simulink model "scen2_PDproposed"  (R2021b)
settings: Solver=ode4  StartTime=0.0  StopTime=tsim+1  FixedStep=sampleRate  RelTol=1e-3
undefined symbols (not defined in the file): alpha, des_x, des_y, des_z, Kd, Kdz, Kp, Kpz, peak_mp, Q, saturation_on, t_end_mp
libraries: dspmtrx3 x1
settings Model: Creator=PC  LastModifiedBy=kangm
settings SolverCC: AlgebraicLoopSolver=TrustRegion
settings DataIOCC: ReturnWorkspaceOutputs=off
settings DebuggingCC: SFMachineParentedDataDiag=warning

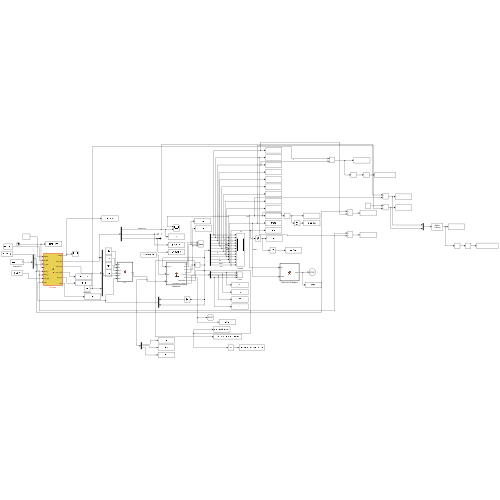
[thumbnail: Simulink's stored preview of the top-level diagram]
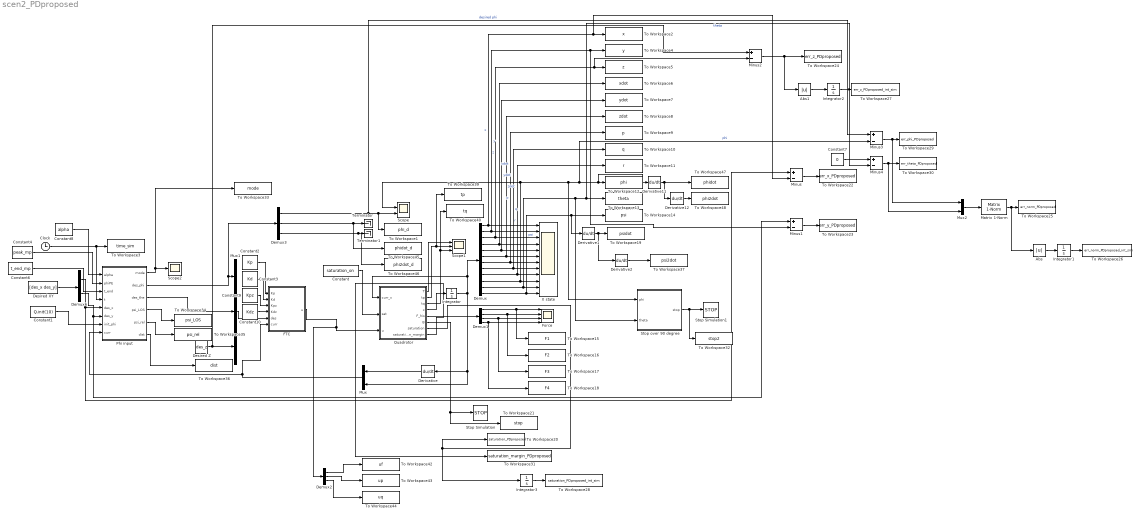
== system scen2_PDproposed ==
  Abs : Abs
  Abs1 : Abs
  Clock : Clock
  Constant : Constant  Value=saturation_on
  Constant1 : Constant  Value=Q.init(10)
  Constant10 : Constant  Value=Kdz
  Constant2 : Constant  Value=Kp
  Constant3 : Constant  Value=Kd
  Constant4 : Constant  Value=peak_mp
  Constant6 : Constant  Value=t_end_mp
  Constant7 : Constant  Value=0
  Constant8 : Constant  Value=alpha
  Constant9 : Constant  Value=Kpz
  Demux : Demux  Outputs=12
  Demux1 : Demux
  Demux2 : Demux  Outputs=3
  Demux3 : Demux  Outputs=3
  Demux6 : Demux  Outputs=2
  Derivative{,1..2,11..12} (5 alike) : Derivative
  Desired XY : Constant  Value=[des_x des_y]
  Desired Z : Constant  Value=des_z
  FTC : MATLAB Function  TreatAsAtomicUnit=on
  Force : Scope  NumInputPorts=4
  Integrator : Integrator  InitialCondition=Q.init
  Integrator1 : Integrator
  Integrator2 : Integrator
  Integrator3 : Integrator
  Matrix 1-Norm : dspmtrx3/Matrix  1-Norm  roundingMode=Floor  overflowMode=off  outputDataTypeStr=Inherit: Same as accumulator  outputMin=[]  outputMax=[]  outputLastDataTypeStr=Inherit: Same as accumulator
      settings: SourceProductBaseCode=DS
  Minus{,1..4} (5 alike) : Sum  Inputs=+-
  Mux : Mux  Inputs=2
  Mux1 : Mux  Inputs=3
  Mux2 : Mux  Inputs=2
  Phi input : MATLAB Function  TreatAsAtomicUnit=on
  Quadrotor : MATLAB Function  TreatAsAtomicUnit=on
  Scope : Scope  NumInputPorts=2
  Scope1 : Scope  NumInputPorts=3
  Scope2 : Scope
  Stop Simulation : Stop
  Stop Simulation1 : Stop
  Stop over 90 degree : MATLAB Function  TreatAsAtomicUnit=on
  Terminator : Terminator
  Terminator1 : Terminator
  To Workspace1 : ToWorkspace  VariableName=phi_d  SampleTime=-1
      settings: Save2DSignal=2-D array (concatenate along first dimension)
  To Workspace10 : ToWorkspace  VariableName=q  SampleTime=-1
      settings: Save2DSignal=2-D array (concatenate along first dimension)
  To Workspace11 : ToWorkspace  VariableName=r  SampleTime=-1
      settings: Save2DSignal=2-D array (concatenate along first dimension)
  To Workspace12 : ToWorkspace  VariableName=phi  SampleTime=-1
      settings: Save2DSignal=2-D array (concatenate along first dimension)
  To Workspace13 : ToWorkspace  VariableName=theta  SampleTime=-1
      settings: Save2DSignal=2-D array (concatenate along first dimension)
  To Workspace14 : ToWorkspace  VariableName=psi  SampleTime=-1
      settings: Save2DSignal=2-D array (concatenate along first dimension)
  To Workspace15 : ToWorkspace  VariableName=F1  SampleTime=-1
      settings: Save2DSignal=2-D array (concatenate along first dimension)
  To Workspace16 : ToWorkspace  VariableName=F2  SampleTime=-1
      settings: Save2DSignal=2-D array (concatenate along first dimension)
  To Workspace17 : ToWorkspace  VariableName=F3  SampleTime=-1
      settings: Save2DSignal=2-D array (concatenate along first dimension)
  To Workspace18 : ToWorkspace  VariableName=F4  SampleTime=-1
      settings: Save2DSignal=2-D array (concatenate along first dimension)
  To Workspace19 : ToWorkspace  VariableName=psidot  SampleTime=-1
      settings: Save2DSignal=2-D array (concatenate along first dimension)
  To Workspace2 : ToWorkspace  VariableName=x  SampleTime=-1
      settings: Save2DSignal=2-D array (concatenate along first dimension)
  To Workspace20 : ToWorkspace  VariableName=saturation_PDproposed  SampleTime=-1
      settings: Save2DSignal=2-D array (concatenate along first dimension)
  To Workspace21 : ToWorkspace  VariableName=stop  SampleTime=-1
      settings: Save2DSignal=2-D array (concatenate along first dimension)
  To Workspace22 : ToWorkspace  VariableName=err_x_PDproposed  SampleTime=-1
      settings: Save2DSignal=2-D array (concatenate along first dimension)
  To Workspace23 : ToWorkspace  VariableName=err_y_PDproposed  SampleTime=-1
      settings: Save2DSignal=2-D array (concatenate along first dimension)
  To Workspace24 : ToWorkspace  VariableName=err_z_PDproposed  SampleTime=-1
      settings: Save2DSignal=2-D array (concatenate along first dimension)
  To Workspace25 : ToWorkspace  VariableName=err_norm_PDproposed  SampleTime=-1
      settings: Save2DSignal=2-D array (concatenate along first dimension)
  To Workspace26 : ToWorkspace  VariableName=err_norm_PDproposed_int_sim  SampleTime=-1
      settings: Save2DSignal=2-D array (concatenate along first dimension)
  To Workspace27 : ToWorkspace  VariableName=err_z_PDproposed_int_sim  SampleTime=-1
      settings: Save2DSignal=2-D array (concatenate along first dimension)
  To Workspace28 : ToWorkspace  VariableName=saturation_PDproposed_int_sim  SampleTime=-1
      settings: Save2DSignal=2-D array (concatenate along first dimension)
  To Workspace29 : ToWorkspace  VariableName=err_phi_PDproposed  SampleTime=-1
      settings: Save2DSignal=2-D array (concatenate along first dimension)
  To Workspace3 : ToWorkspace  VariableName=time_sim  SampleTime=-1
      settings: Save2DSignal=2-D array (concatenate along first dimension)
  To Workspace30 : ToWorkspace  VariableName=err_theta_PDproposed  SampleTime=-1
      settings: Save2DSignal=2-D array (concatenate along first dimension)
  To Workspace31 : ToWorkspace  VariableName=saturation_margin_PDproposed  SampleTime=-1
      settings: Save2DSignal=2-D array (concatenate along first dimension)
  To Workspace32 : ToWorkspace  VariableName=stop2  SampleTime=-1
      settings: Save2DSignal=2-D array (concatenate along first dimension)
  To Workspace33 : ToWorkspace  VariableName=mode  SampleTime=-1
      settings: Save2DSignal=2-D array (concatenate along first dimension)
  To Workspace34 : ToWorkspace  VariableName=psi_LOS  SampleTime=-1
      settings: Save2DSignal=2-D array (concatenate along first dimension)
  To Workspace35 : ToWorkspace  VariableName=psi_rel  SampleTime=-1
      settings: Save2DSignal=2-D array (concatenate along first dimension)
  To Workspace36 : ToWorkspace  VariableName=dist  SampleTime=-1
      settings: Save2DSignal=2-D array (concatenate along first dimension)
  To Workspace37 : ToWorkspace  VariableName=psi2dot  SampleTime=-1
      settings: Save2DSignal=2-D array (concatenate along first dimension)
  To Workspace39 : ToWorkspace  VariableName=tp  SampleTime=-1
      settings: Save2DSignal=2-D array (concatenate along first dimension)
  To Workspace4 : ToWorkspace  VariableName=y  SampleTime=-1
      settings: Save2DSignal=2-D array (concatenate along first dimension)
  To Workspace40 : ToWorkspace  VariableName=tq  SampleTime=-1
      settings: Save2DSignal=2-D array (concatenate along first dimension)
  To Workspace42 : ToWorkspace  VariableName=uf  SampleTime=-1
      settings: Save2DSignal=2-D array (concatenate along first dimension)
  To Workspace43 : ToWorkspace  VariableName=up  SampleTime=-1
      settings: Save2DSignal=2-D array (concatenate along first dimension)
  To Workspace44 : ToWorkspace  VariableName=uq  SampleTime=-1
      settings: Save2DSignal=2-D array (concatenate along first dimension)
  To Workspace45 : ToWorkspace  VariableName=phidot_d  SampleTime=-1
      settings: Save2DSignal=2-D array (concatenate along first dimension)
  To Workspace46 : ToWorkspace  VariableName=phi2dot_d  SampleTime=-1
      settings: Save2DSignal=2-D array (concatenate along first dimension)
  To Workspace47 : ToWorkspace  VariableName=phidot  SampleTime=-1
      settings: Save2DSignal=2-D array (concatenate along first dimension)
  To Workspace48 : ToWorkspace  VariableName=phi2dot  SampleTime=-1
      settings: Save2DSignal=2-D array (concatenate along first dimension)
  To Workspace5 : ToWorkspace  VariableName=z  SampleTime=-1
      settings: Save2DSignal=2-D array (concatenate along first dimension)
  To Workspace6 : ToWorkspace  VariableName=xdot  SampleTime=-1
      settings: Save2DSignal=2-D array (concatenate along first dimension)
  To Workspace7 : ToWorkspace  VariableName=ydot  SampleTime=-1
      settings: Save2DSignal=2-D array (concatenate along first dimension)
  To Workspace8 : ToWorkspace  VariableName=zdot  SampleTime=-1
      settings: Save2DSignal=2-D array (concatenate along first dimension)
  To Workspace9 : ToWorkspace  VariableName=p  SampleTime=-1
      settings: Save2DSignal=2-D array (concatenate along first dimension)
  X state : Scope  NumInputPorts=12
  wires:
  Quadrotor/4(x) -> Integrator/1
  Mux1/1 -> FTC/5(des)
  Integrator/1 -> Demux/1, Quadrotor/1(curr_x), Derivative/1, Mux/2
  Demux/1 -> Minus/2, To Workspace2/1, X state/1  "x"
  Demux/2 -> Minus1/2, To Workspace4/1, X state/2  "y"
  Demux/4 -> To Workspace6/1, X state/4  "xdot"
  Demux/5 -> To Workspace7/1, X state/5  "ydot"
  Demux/6 -> To Workspace8/1, X state/6  "zdot"
  Demux/7 -> To Workspace9/1, X state/7  "p"
  Demux/8 -> To Workspace10/1, X state/8  "q"
  Demux/9 -> To Workspace11/1, X state/9  "r"
  Mux/1 -> FTC/6(curr), Phi input/8(curr)
  Derivative/1 -> Mux/1
  Clock/1 -> Phi input/4(t), To Workspace3/1
  Demux6/1 -> Minus/1, Phi input/5(des_x)
  Desired XY/1 -> Demux6/1
  Quadrotor/5(F_his) -> Demux1/1
  Demux1/1 -> Force/1, To Workspace15/1
  Demux1/3 -> Force/3, To Workspace17/1
  Demux1/4 -> Force/4, To Workspace18/1
  Demux1/2 -> Force/2, To Workspace16/1
  Demux/12 -> Derivative1/1, To Workspace14/1, X state/12  "psi"
  Derivative1/1 -> Derivative2/1, To Workspace19/1
  Constant/1 -> Quadrotor/2(sat)
  Demux3/3 -> To Workspace46/1, Terminator1/1
  Constant1/1 -> Phi input/7(init_phi)
  Phi input/2(des_phi) -> Demux3/1, Mux1/1
  Phi input/3(des_the) -> Mux1/2
  Constant6/1 -> Phi input/3(t_end)
  Constant4/1 -> Phi input/2(phiPE)
  Constant2/1 -> FTC/1(Kp)
  Constant3/1 -> FTC/2(Kd)
  Quadrotor/1(T) -> Scope1/1
  Quadrotor/6(B) -> To Workspace21/1, Stop Simulation/1
  Quadrotor/7(saturation) -> To Workspace20/1, Integrator3/1
  Integrator3/1 -> To Workspace28/1
  Demux/3 -> Minus2/2, To Workspace5/1, X state/3  "z"
  Minus1/1 -> To Workspace23/1
  Demux6/2 -> Minus1/1, Phi input/6(des_y)
  Matrix 1-Norm/1 -> Abs/1, To Workspace25/1
  Demux3/1 -> To Workspace1/1, Scope/2, Minus3/1  "desired phi"
  Mux2/1 -> Matrix 1-Norm/1
  Desired Z/1 -> Minus2/1, Mux1/3
  Abs/1 -> Integrator1/1
  Integrator1/1 -> To Workspace26/1
  Abs1/1 -> Integrator2/1
  Integrator2/1 -> To Workspace27/1
  Minus/1 -> To Workspace22/1
  Minus2/1 -> Abs1/1, To Workspace24/1
  Minus3/1 -> Mux2/1, To Workspace29/1
  Minus4/1 -> Mux2/2, To Workspace30/1
  Constant7/1 -> Minus4/1
  Demux/10 -> Stop over 90 degree/1(phi), Minus3/2, Derivative11/1, To Workspace12/1, Scope/1, X state/10  "phi"
  Stop over 90 degree/1(stop) -> To Workspace32/1, Stop Simulation1/1
  Demux/11 -> Stop over 90 degree/2(theta), Minus4/2, To Workspace13/1, X state/11  "theta"
  Quadrotor/8(saturation_margin) -> To Workspace31/1
  Phi input/1(mode) -> To Workspace33/1, Scope2/1
  Derivative2/1 -> To Workspace37/1
  Demux3/2 -> To Workspace45/1, Terminator/1
  Phi input/4(psi_LOS) -> To Workspace34/1
  Phi input/5(psi_rel) -> To Workspace35/1
  Phi input/6(dist) -> To Workspace36/1
  Quadrotor/3(tq) -> To Workspace40/1, Scope1/3
  Quadrotor/2(tp) -> To Workspace39/1, Scope1/2
  Demux2/3 -> To Workspace44/1
  Demux2/2 -> To Workspace43/1
  Demux2/1 -> To Workspace42/1
  FTC/1(u) -> Demux2/1, Quadrotor/3(u)
  Derivative11/1 -> Derivative12/1, To Workspace47/1
  Derivative12/1 -> To Workspace48/1
  Constant8/1 -> Phi input/1(alpha)
  Constant10/1 -> FTC/4(Kdz)
  Constant9/1 -> FTC/3(Kpz)

== matlab function scen2_PDproposed/FTC ==
  data: Kp input; Kd input; Kpz input; Kdz input; des input; u output; curr input
function u   = pd(Kp,Kd,Kpz,Kdz,des,curr)

m = 1.282; g = 9.81;
Ix = 4.856*10^-3; Iy = Ix; Iz = 8.801*10^-3;
b = 0.0066;
kr = 0.02; %drag coefficient
kt = 0.5;
% kt = 0.25;
l = 0.1;

% current state
N = 0;
xdot   = curr(N+1); ydot   = curr(N+2); zdot   = curr(N+3);
x2dot  = curr(N+4); y2dot  = curr(N+5); z2dot  = curr(N+6);
pdot   = curr(N+7); qdot   = curr(N+8); rdot   = curr(N+9);
phidot = curr(N+10);thedot = curr(N+11);psidot = curr(N+12);

N = 12;
x    = curr(N+1); y    = curr(N+2); z    = curr(N+3);
xdot = curr(N+4); ydot = curr(N+5); zdot = curr(N+6);
p    = curr(N+7); q    = curr(N+8); r    = curr(N+9);
phi  = curr(N+10);the  = curr(N+11);psi  = curr(N+12);
des_temp = zeros(7,1);
des_temp = des;
des = des_temp;
% desired state
phi_d = des(1);
phidot_d = des(2);
phi2dot_d = des(3);
the_d = des(4);
thedot_d = des(5);
the2dot_d = des(6);
z_d   = des(7);


% Feedback PD Control
% phi
% phi2dot = f1(~~)+1/Ix*tp

% Kp = 3;
% Kd = 4;

% Kp = 100;
% Kd = 1;

F = [p + q*sin(phi)*tan(the) + r*cos(phi)*tan(the)
     q*cos(phi) - r*sin(phi)
     -(Iz - Iy)*q*r/Ix
     -(Ix - Iz)*p*r/Iy
     -kr*r/Iz
     zdot
     -kt*zdot/m - g];
 
G = [0 0 0
     0 0 0
     0 1/Ix 0
     0 0 1/Iy
     b/Iz -2*b/(l*Iz) 0
     0 0 0
     cos(phi)*cos(the)/m 0 0];
 
J = [q*cos(phi)*tan(the)-r*sin(phi)*tan(the) q*sin(phi)*sec(the)^2+r*cos(phi)*sec(the)^2 1 sin(phi)*tan(the) cos(phi)*tan(the) 0 0
     -q*sin(phi)-r*cos(phi) 0 0 cos(phi) -sin(phi) 0 0
     0 0 0 0 0 0 1];

ubar = [phi2dot_d + Kp*(phi_d-phi) + Kd*(phidot_d-phidot)
        the2dot_d + Kp*(the_d-the) + Kd*(thedot_d-thedot)
        Kpz*(z_d-z) + Kdz*(0-zdot)];
    
u = inv(J*G)*(-J*F + ubar);

% u = [12.5813 0.0013 0]';
% u = [13.3835 0.0259 0]';

% tp = u_prev(1);
% tq = u_prev(2);
% T = u_prev(3);

 
% f1 = qdot*sin(phi)*tan(the) + q*cos(phi)*phidot*tan(the) + q*sin(phi)*1/cos(the)^2*thedot...
%     + rdot*cos(phi)*tan(the) + r*(-sin(phi)*phidot)*tan(the) + r*cos(phi)*1/cos(the)^2*thedot ...
%     + (Ix-Iz)/Ix*q*r;
% 
% % tp = Ix*(-f1+ 3*(phi_d-phi) + 4*(phidot_d-phidot));
% tp = Ix*(-f1+ Kp*(phi_d-phi) + Kd*(phidot_d-phidot));
% 
% 
% %theta
% %the2dot = g1(~~) + cos(phi)/Ix * tq
% h1 = -q*sin(phi)*phidot-rdot*sin(phi)-r*cos(phi)*phidot ...
%     + (Iz-Ix)/Ix*p*r*cos(phi);
% % tq = Ix*(-h1+ 3*(the_d-the) + 5*(thedot_d-thedot));
% tq = Ix*(-h1+ Kp*(the_d-the) + Kd*(thedot_d-thedot));
% 
% %z
% T = m/(cos(the)*cos(phi))*(g + 3*(z_d-z) + (0-zdot));

% u = [T tp tq]';

== matlab function scen2_PDproposed/Quadrotor ==
  data: T output; tp output; tq output; curr_x input; sat input; u input; x output; F_his output; B output; saturation output; saturation_margin output
function [T,tp,tq,x,F_his,B,saturation,saturation_margin] = system(curr_x,sat,u)
% x = {xyz xyzvel pqr phi theta psi}
x = zeros(12,1);
% Properties
m = 1.282; g = 9.81;
Ix = 4.856*10^-3; Iy = Ix; Iz = 8.801*10^-3;
b = 0.0066;
kr = 0.02;
kt = 0.5;
l = 0.1;

u_temp = zeros(3,1);
u_temp = u;
u = u_temp;

T = u(1); tp = u(2); tq = u(3);% tr = u(4);
tr = b*(T-2*tp/l);
A = [1 1 1; 0 l 0;-l 0 l];

F=inv(A)*[T tp tq]';

f1 = F(1); f2 = F(2); f3 = F(3);
ub = m*g;
lb = 0;

saturation1_lb = 0;
saturation1_ub = 0;
saturation2_lb = 0;
saturation2_ub = 0;
saturation3_lb = 0;
saturation3_ub = 0;
saturation1_lb_margin = 0;
saturation1_ub_margin = 0;
saturation2_lb_margin = 0;
saturation2_ub_margin = 0;
saturation3_lb_margin = 0;
saturation3_ub_margin = 0;

if sat == 1
    if f1 < lb
        saturation1_lb = abs(lb - f1);
        saturation1_lb_margin = abs(lb - f1);
        f1 = lb;
    else
        saturation1_lb_margin = lb - f1;
    end
    
    if f1 > ub
        saturation1_ub = abs(ub - f1);
        saturation1_ub_margin = abs(ub - f1);
        f1 = ub;
    else
        saturation1_ub_margin = f1 - ub;
    end
    
    if f2 < lb
        saturation2_lb = abs(lb - f2);
        saturation2_lb_margin = abs(lb - f2);
        f2 = lb;
    else
        saturation2_lb_margin = lb - f2;
    end
    
    if f2 > ub
        saturation2_ub = abs(ub - f2);
        saturation2_ub_margin = abs(ub - f2);
        f2 = ub;
    else
        saturation2_ub_margin = f2 - ub;
    end
    
    if f3 < lb
        saturation3_lb = abs(lb - f3);
        saturation3_lb_margin = abs(lb - f3);
        f3 = lb;
    else
        saturation3_lb_margin = lb - f3;
    end
    
    if f3 > ub
        saturation3_ub = abs(ub - f3);
        saturation3_ub_margin = abs(ub - f3);
        f3 = ub;
    else
        saturation3_ub_margin = f3 - ub;
    end
end

saturation = max([saturation1_lb,saturation1_ub,saturation2_lb,saturation2_ub,saturation3_lb,saturation3_ub]);
saturation_margin = max([saturation1_lb_margin,saturation1_ub_margin,saturation2_lb_margin,saturation2_ub_margin,saturation3_lb_margin,saturation3_ub_margin]);

f4 = 0;
F_his = [f1 f2 f3 f4]';
T = f1+f2+f3;
tp = l*(f2);
tq = l*(f3-f1);
tr = b*(f1+f3-f2);

% Current state
x1  = curr_x(1);
x2  = curr_x(2);
x3  = curr_x(3);
x4  = curr_x(4);
x5  = curr_x(5);
x6  = curr_x(6);
x7  = curr_x(7);
x8  = curr_x(8);
x9  = curr_x(9);
x10 = curr_x(10);
x11 = curr_x(11);
x12 = curr_x(12);

% Position
x(1) = x4;
x(2) = x5;
x(3) = x6;
% Velocity
x(4) = T/m*(cos(x12)*sin(x11)*cos(x10) + sin(x12)*sin(x10)) - kt/m*x4;
x(5) = T/m*(sin(x12)*sin(x11)*cos(x10) - cos(x12)*sin(x10)) - kt/m*x5;
x(6) = -g + T*(1/m)*(cos(x10)*cos(x11)) - kt/m*x6;
% Body rate
x(7) = ((Ix-Iz)*x8*x9 + tp)/Ix;
x(8) = ((Iz-Ix)*x7*x9 + tq)/Ix;
x(9) = (-kr*x9 + tr)/Iz;
% Angle
x(10) = x7 + x8*sin(x10)*tan(x11) + x9*cos(x10)*tan(x11);
x(11) = x8*cos(x10) - x9*sin(x10);
x(12) = x8*sin(x10)/cos(x11) + x9*cos(x10)*cos(x11);

if x3<=0
    B=1;
else
    B=0;
end

== matlab function scen2_PDproposed/Stop over 90 degree ==
  data: phi input; stop output; theta input
function stop = fcn(phi, theta)

stop = 0;
max_attitude = deg2rad(90);

if abs(phi) >= max_attitude || abs(theta) >= max_attitude
    stop = 1;
end

== matlab function scen2_PDproposed/Phi input ==
  settings: updateMethod=DISCRETE
  data: alpha input; mode output; phiPE input; t_end input; des_phi output; des_the output; t input; des_x input; des_y input; init_phi input; curr input; psi_LOS output; psi_rel output; dist output
function [mode,des_phi,des_the,psi_LOS,psi_rel,dist]  = fcn(alpha,phiPE,t_end,t,des_x,des_y,init_phi,curr)

m = 1.282; g = 9.81;
Ix = 4.856*10^-3; Iz = 8.801*10^-3; Iy = Ix; I = (Iz-Iy)/Ix;
b = 0.0066;
kr = 0.02; %drag coefficient
kt = 0.5;
l = 0.1;

phi0 = init_phi;
T = t_end;

rPE = (-kr/b+sqrt((kr/b)^2+8*m*g/(l*cos(phiPE))*(Iz-Iy)*tan(phiPE)))/(4*(Iz-Iy)*tan(phiPE)/l);
psidotPE = rPE*(tan(phiPE)*sin(phiPE)+cos(phiPE)); 
TPE = 2*pi/psidotPE;

phiPE2 = phiPE - alpha;
rPE2 = (-kr/b+sqrt((kr/b)^2+8*m*g/(l*cos(phiPE2))*(Iz-Iy)*tan(phiPE2)))/(4*(Iz-Iy)*tan(phiPE2)/l);
psidotPE2 = rPE2*(tan(phiPE2)*sin(phiPE2)+cos(phiPE2)); 
TPE2 = 2*pi/psidotPE2;

fPE2 = 1/TPE2;
fPE2 = fPE2*1.0004;
toff = 1/(4*fPE2);

a0 = phi0;
a1 = 0;
a2 = 0;
a3 = - (10*phi0 - 10*phiPE)/T^3;
a4 = (15*phi0 - 15*phiPE)/T^4;
a5 = -(6*phi0 - 6*phiPE)/T^5;

% current state
N = 0;
xdot   = curr(N+1); ydot   = curr(N+2); zdot   = curr(N+3);
x2dot  = curr(N+4); y2dot  = curr(N+5); z2dot  = curr(N+6);
pdot   = curr(N+7); qdot   = curr(N+8); rdot   = curr(N+9);
phidot = curr(N+10);thedot = curr(N+11);psidot = curr(N+12);

N = 12;
x    = curr(N+1); y    = curr(N+2); z    = curr(N+3);
xdot = curr(N+4); ydot = curr(N+5); zdot = curr(N+6);
p    = curr(N+7); q    = curr(N+8); r    = curr(N+9);
phi  = curr(N+10);the  = curr(N+11);psi  = curr(N+12);

while psi > pi
    psi = psi - 2*pi;
end

while psi < -pi
    psi = psi + 2*pi;
end

R = 0.2016;

C_x = des_x;
C_y = des_y;
x_d = -R*sin(psi) + C_x; y_d = R*cos(psi) + C_y;
xdot_d = -R*cos(psi)*psidot; ydot_d = -R*sin(psi)*psidot;

dist = sqrt((x_d-x)^2+(y_d-y)^2);

psi_LOS = atan2(des_y-y,des_x-x);

psi_rel = psi_LOS - psi;
while psi_rel > pi
    psi_rel = psi_rel - 2*pi;
end

while psi_rel < -pi
    psi_rel = psi_rel + 2*pi;
end

kp = 1; kd = 1.5;

persistent x0 y0 psi0 psi_LOS0 xPSMP yPSMP psiPSMP tPSMP tauPSMP 
if isempty(x0)
    x0 = 0;
end
if isempty(y0)
    y0 = 0;
end
if isempty(psi0)
    psi0 = 0;
end
if isempty(psi_LOS0)
    psi_LOS0 = 0;
end
if isempty(xPSMP)
    xPSMP = 0;
end
if isempty(yPSMP)
    yPSMP = 0;
end
if isempty(psiPSMP)
    psiPSMP = 0;
end
if isempty(tPSMP)
    tPSMP = 0;
end
if isempty(tauPSMP)
    tauPSMP = 0;
end

data = [x0,y0,psi0,xPSMP,yPSMP,psiPSMP,psi_LOS0,tauPSMP,tPSMP];

delay_gain = 15;

% Obtained by ASMP,
% phi_hat = 0.6974;
phi_d = 0;
phidot_d = 0;
phi2dot_d = 0;

attitude_error_margin = deg2rad(1);

mode = 0;

switch_psi = 0;
switch_pos = 0;

persistent switch_psi_occ
if isempty(switch_psi_occ)
    switch_psi_occ = 0;
end

persistent switch_pos_occ
if isempty(switch_pos_occ)
    switch_pos_occ = 0;
end

% Motion planner
if t <= t_end
    phi_d = a0 + a1*t + a2*t^2 + a3*t^3 + a4*t^4 + a5*t^5;
    phidot_d = a1 + 2*a2*t + 3*a3*t^2 + 4*a4*t^3 + 5*a5*t^4;
    phi2dot_d = 2*a2 + 6*a3*t + 12*a4*t^2 + 20*a5*t^3;
elseif t <= t_end*delay_gain
    phi_d = phiPE;
    phidot_d = 0;
    phi2dot_d = 0;
    x0 = x;
    y0 = y;
    psi0 = psi;
    psi_LOS0 = atan2(des_y-y0,des_x-x0);
    tauPSMP = (psi_LOS0-psi0-pi-psidotPE2*toff)/psidotPE + 0.035;
    while tauPSMP < 0
        tauPSMP = tauPSMP + TPE;
    end
    tPSMP = t_end*delay_gain + tauPSMP;
elseif t <= t_end*delay_gain + tauPSMP % *0.98
    phi_d = phiPE;
    phidot_d = 0;
    phi2dot_d = 0;
    xPSMP = x;
    yPSMP = y;
    psiPSMP = psi;
else
    % PSMP
    phi_d = phiPE + alpha*(-sin(2*pi*fPE2*(t-1/(4*fPE2)-tPSMP)) - 1); % Down
    phidot_d = -2*alpha*pi*fPE2*cos(2*pi*fPE2*(t-1/(4*fPE2)-tPSMP));
    phi2dot_d = 4*alpha*(pi*fPE2)^2*sin(2*pi*fPE2*(t-1/(4*fPE2)-tPSMP));

    mode = 2;
    switch_psi_occ = 1;
end

the_d = 0;    
thedot_d = 0;
the2dot_d = 0;

des_phi = [phi_d, phidot_d, phi2dot_d]';
des_the = [the_d, thedot_d, the2dot_d]';
